simulink library "outputHandlingSubsytem"  (R2021b)
settings: Solver=VariableStepAuto  StartTime=0.0  StopTime=10.0  RelTol=1e-3
settings Model: Creator=mat  LastModifiedBy=mat

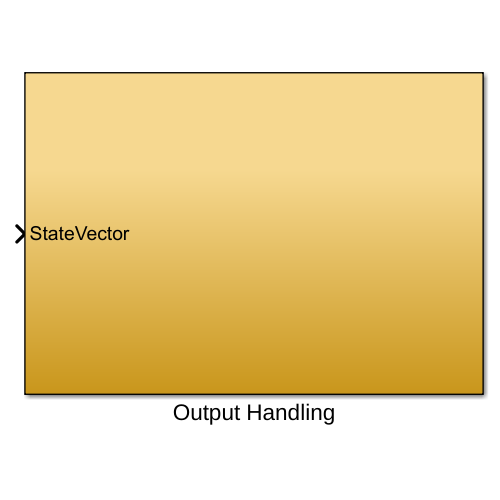
[thumbnail: Simulink's stored preview of the top-level diagram]
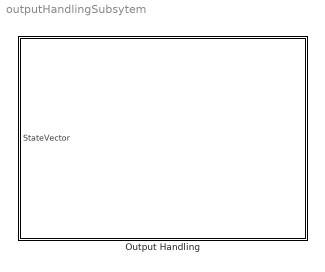
== system outputHandlingSubsytem ==
  Output Handling : Subsystem

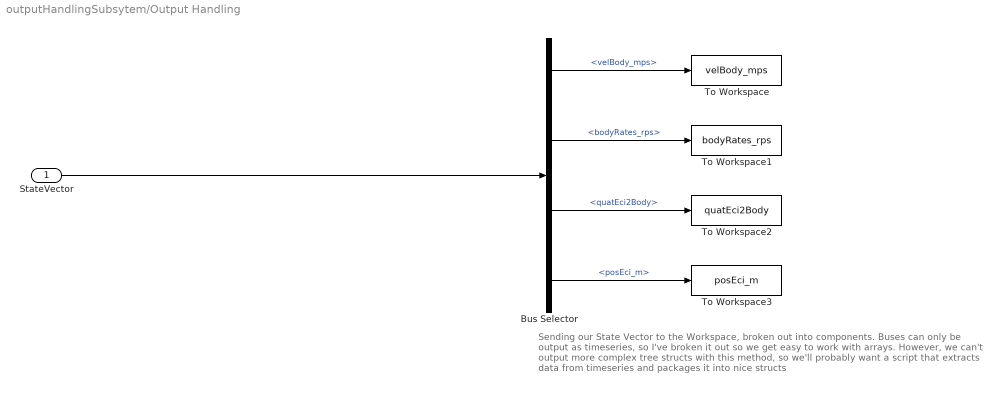
== system outputHandlingSubsytem/Output Handling ==
  note: Sending our State Vector to the Workspace, broken out into components. Buses can only be output as timeseries, so I've broken it out so we get easy to work with arrays. However, we can't output more complex tree structs with this method, so we'll probably want a script that extracts data from timeseries and packages it into nice structs
  StateVector : Inport  OutDataTypeStr=Bus: StateVector_BusType
  Bus Selector : BusSelector  OutputSignals=velBody_mps,bodyRates_rps,quatEci2Body,posEci_m
  To Workspace : ToWorkspace  VariableName=velBody_mps  SampleTime=-1
      settings: Save2DSignal=2-D array (concatenate along first dimension)
  To Workspace1 : ToWorkspace  VariableName=bodyRates_rps  SampleTime=-1
      settings: Save2DSignal=2-D array (concatenate along first dimension)
  To Workspace2 : ToWorkspace  VariableName=quatEci2Body  SampleTime=-1
      settings: Save2DSignal=2-D array (concatenate along first dimension)
  To Workspace3 : ToWorkspace  VariableName=posEci_m  SampleTime=-1
      settings: Save2DSignal=2-D array (concatenate along first dimension)
  wires:
  Bus Selector/2 -> To Workspace1/1  "<bodyRates_rps>"
  Bus Selector/1 -> To Workspace/1  "<velBody_mps>"
  Bus Selector/3 -> To Workspace2/1  "<quatEci2Body>"
  StateVector/1 -> Bus Selector/1
  Bus Selector/4 -> To Workspace3/1  "<posEci_m>"
